simulink model "FIR_filter_direct_form"  (R2020b)
settings: Solver=VariableStepAuto  StartTime=0.0  StopTime=10.0  RelTol=1e-3
model workspace (MAT data in the model file):
  a1 = 2
  a2 = -3
  a3 = -4
  a4 = 5
settings Model: Creator=user  LastModifiedBy=user

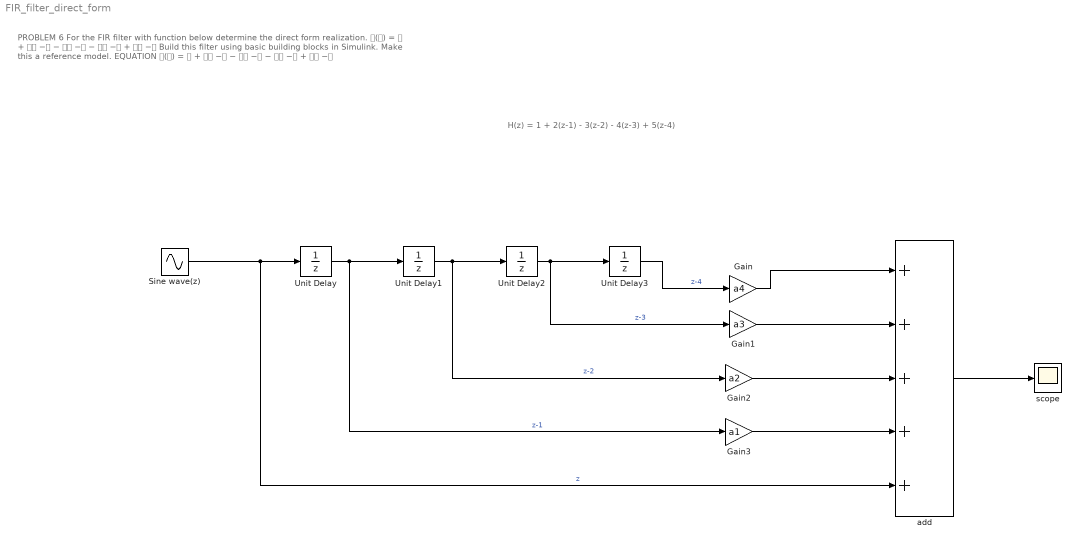
== system FIR_filter_direct_form ==
  note: H(z) = 1 + 2(z-1) - 3(z-2) - 4(z-3) + 5(z-4)
  note: PROBLEM 6
      |
      | For the FIR filter with function below determine the direct form realization. 𝐇(𝐳) = 𝟏 + 𝟐𝐳 −𝟏 − 𝟑𝐳 −𝟐 − 𝟒𝐳 −𝟑 + 𝟓𝐳 −𝟒 Build this filter using basic building blocks in Simulink. Make this a reference model.
      |
      | EQUATION
      | 𝐇(𝐳) = 𝟏 + 𝟐𝐳 −𝟏 − 𝟑𝐳 −𝟐 − 𝟒𝐳 −𝟑 + 𝟓𝐳 −𝟒
  Gain : Gain  Gain=a4
  Gain1 : Gain  Gain=a3
  Gain2 : Gain  Gain=a2
  Gain3 : Gain  Gain=a1
  Sine wave(z) : Sin  SampleTime=0
  Unit Delay{,1..3} (4 alike) : UnitDelay  SampleTime=-1  HasFrameUpgradeWarning=on
  add : Sum  Inputs=+++++
  scope : Scope
  wires:
  Sine wave(z)/1 -> add/5, Unit Delay/1  "z"
  Unit Delay/1 -> Gain3/1, Unit Delay1/1  "z-1"
  Unit Delay1/1 -> Gain2/1, Unit Delay2/1  "z-2"
  Unit Delay2/1 -> Gain1/1, Unit Delay3/1  "z-3"
  Unit Delay3/1 -> Gain/1  "z-4"
  Gain/1 -> add/1
  Gain2/1 -> add/3
  add/1 -> scope/1
  Gain3/1 -> add/4
  Gain1/1 -> add/2
